simulink model "DroneForwardingSimulation"  (R2022b)
settings: Solver=ode45  StartTime=0.0  StopTime=60  MaxStep=0.2  RelTol=1e-4  AbsTol=1e-4
libraries: slpidlib x2
settings Model: Creator=aless  LastModifiedBy=aless

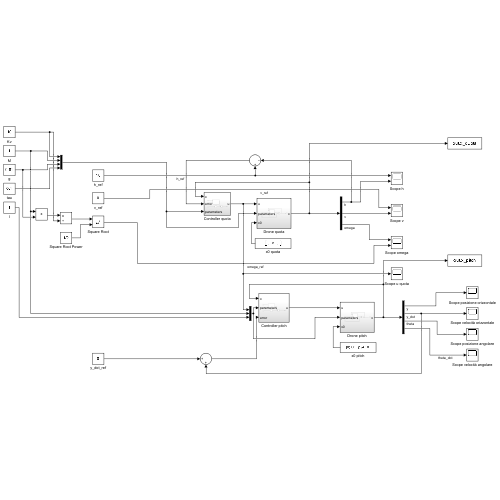
[thumbnail: Simulink's stored preview of the top-level diagram]
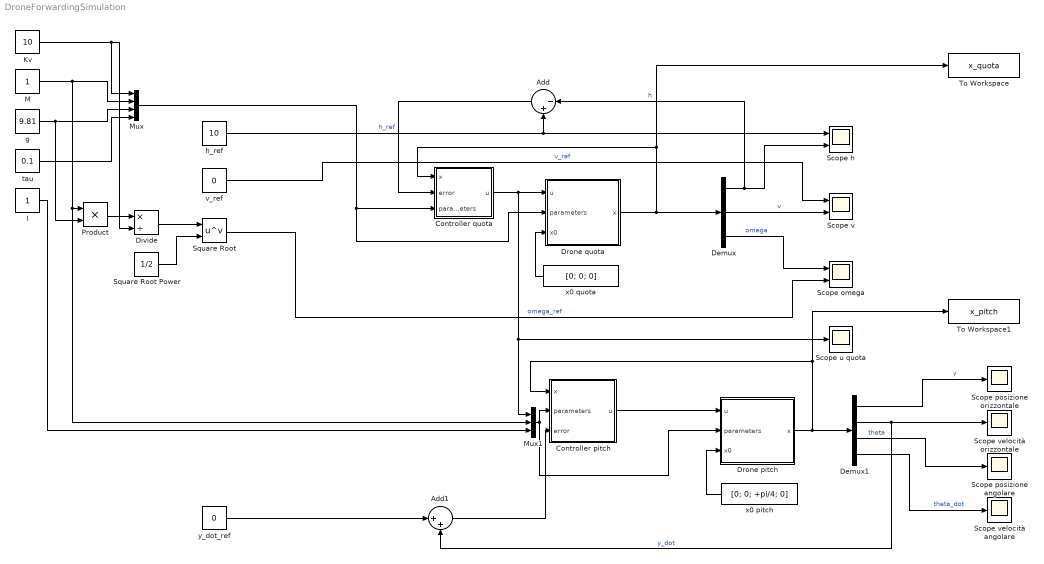
== system DroneForwardingSimulation ==
  Add : Sum  Inputs=|-+
  Add1 : Sum  Inputs=|++
  Controller pitch : Subsystem
  Controller quota : Subsystem
  Demux : Demux  Outputs=3
  Demux1 : Demux
  Divide : Product  Inputs=*/
  Drone pitch : Subsystem
  Drone quota : Subsystem
  I : Constant
  Kv : Constant  Value=10
  M : Constant
  Mux : Mux
  Mux1 : Mux  Inputs=3
  Product : Product
  Scope h : Scope  NumInputPorts=2
  Scope omega : Scope  NumInputPorts=2
  Scope posizione angolare : Scope
  Scope posizione orizzontale : Scope
  Scope u quota : Scope
  Scope v : Scope  NumInputPorts=2
  Scope velocità angolare : Scope
  Scope velocità orizzontale : Scope
  Square Root : Math  Operator=pow
  Square Root Power : Constant  Value=1/2
  To Workspace : ToWorkspace  VariableName=x_quota  SaveFormat=Timeseries  SampleTime=-1
  To Workspace1 : ToWorkspace  VariableName=x_pitch  SaveFormat=Timeseries  SampleTime=-1
  g : Constant  Value=9.81
  h_ref : Constant  Value=10
  tau : Constant  Value=0.1
  v_ref : Constant  Value=0
  x0 pitch : Constant  Value=[0; 0; +pi/4; 0]
  x0 quota : Constant  Value=[0; 0; 0]
  y_dot_ref : Constant  Value=0
  wires:
  Drone quota/1(x) -> To Workspace/1, Controller quota/1(x), Demux/1
  Controller quota/1(u) -> Mux1/1, Scope u quota/1, Drone quota/1(u)
  Demux/1 -> Add/1, Scope h/2  "h"
  g/1 -> Product/2, Mux/3
  M/1 -> Mux1/2, Product/1, Mux/2
  Kv/1 -> Divide/2, Mux/1
  tau/1 -> Mux/4
  Demux/2 -> Scope v/2  "v"
  Demux/3 -> Scope omega/1  "omega"
  x0 quota/1 -> Drone quota/3(x0)
  h_ref/1 -> Scope h/1, Add/2  "h_ref"
  Square Root Power/1 -> Square Root/2
  Product/1 -> Divide/1
  Divide/1 -> Square Root/1
  Square Root/1 -> Scope omega/2  "omega_ref"
  v_ref/1 -> Scope v/1  "v_ref"
  Mux/1 -> Drone quota/2(parameters), Controller quota/3(parameters)
  Add/1 -> Controller quota/2(error)
  Controller pitch/1(u) -> Drone pitch/1(u)
  x0 pitch/1 -> Drone pitch/3(x0)
  Mux1/1 -> Drone pitch/2(parameters), Controller pitch/2(parameters)
  Drone pitch/1(x) -> Demux1/1, To Workspace1/1, Controller pitch/1(x)
  I/1 -> Mux1/3
  Demux1/1 -> Scope posizione orizzontale/1  "y"
  Demux1/2 -> Add1/2, Scope velocità orizzontale/1  "y_dot"
  Demux1/3 -> Scope posizione angolare/1  "theta"
  Demux1/4 -> Scope velocità angolare/1  "theta_dot"
  Add1/1 -> Controller pitch/3(error)
  y_dot_ref/1 -> Add1/1

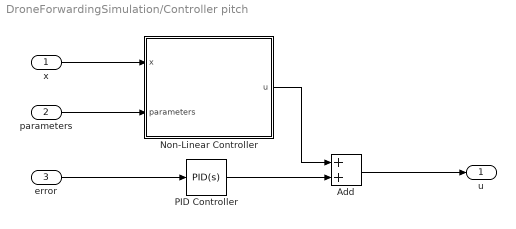
== system DroneForwardingSimulation/Controller pitch ==
  x : Inport
  parameters : Inport  Port=2
  error : Inport  Port=3
  Add : Sum
  Non-Linear Controller : MATLAB Function  TreatAsAtomicUnit=on
  PID Controller : slpidlib/PID Controller  Controller=PID  Form=Parallel  TimeDomain=Continuous-time  UseExternalTs=off  SampleTime=-1  IntegratorMethod=Forward Euler  FilterMethod=Forward Euler  ControllerParametersSource=internal  P=1  I=0.1  UseKiTs=off  D=0  N=100  UseFilter=on  TunerSelectOption=Transfer Function Based (PID Tuner App)  InitialConditionSource=internal  InitialConditionForIntegrator=0  InitialConditionForFilter=0  DifferentiatorICPrevScaledInput=0  ExternalReset=none  TrackingMode=off  Kt=1  LimitOutput=off  SatLimitsSource=internal  UpperSaturationLimit=inf  LowerSaturationLimit=-inf  LinearizeAsGain=on  AntiWindupMode=none  Kb=1  LimitIntegrator=off  UpperIntegratorSaturationLimit=inf  LowerIntegratorSaturationLimit=-inf  POutMin=[]  POutMax=[]  IOutMin=[]  IOutMax=[]  DOutMin=[]  DOutMax=[]  NOutMin=[]  NOutMax=[]  SumOutMin=[]  SumOutMax=[]  SaturationOutMin=[]  SaturationOutMax=[]  PParamMin=[]  PParamMax=[]  IParamMin=[]  IParamMax=[]  DParamMin=[]  DParamMax=[]  NParamMin=[]  NParamMax=[]  KbParamMin=[]  KbParamMax=[]  KtParamMin=[]  KtParamMax=[]  KbOutMin=[]  KbOutMax=[]  KtOutMin=[]  KtOutMax=[]  IntegratorOutMin=[]  IntegratorOutMax=[]  FilterOutMin=[]  FilterOutMax=[]  SumI1OutMin=[]  SumI1OutMax=[]  SumI2OutMin=[]  SumI2OutMax=[]  SumI3OutMin=[]  SumI3OutMax=[]  SumI4OutMin=[]  SumI4OutMax=[]  SumDOutMin=[]  SumDOutMax=[]  DifferentiatorOutMin=[]  DifferentiatorOutMax=[]  FilterDiffOutCoefMin=[]  FilterDiffOutCoefMax=[]  ReciprocalOutMin=[]  ReciprocalOutMax=[]  SumDenOutMin=[]  SumDenOutMax=[]  SumNumOutMin=[]  SumNumOutMax=[]  DivideOutMin=[]  DivideOutMax=[]  UdiffTsProdOutMin=[]  UdiffTsProdOutMax=[]  NTsProdOutMin=[]  NTsProdOutMax=[]  UintegralTsProdOutMin=[]  UintegralTsProdOutMax=[]  UngainTsProdOutMin=[]  UngainTsProdOutMax=[]  ClampingZeroOutDataTypeStr=Inherit: Inherit via back propagation  ClampingZeroOutMin=[]  ClampingZeroOutMax=[]  FilterDenConstantOutDataTypeStr=Inherit: Inherit via back propagation  FilterDenConstantOutMin=[]  FilterDenConstantOutMax=[]  PCopyOutDataTypeStr=Inherit: Inherit via back propagation  PCopyOutMin=[]  PCopyOutMax=[]  NCopyOutDataTypeStr=Inherit: Inherit via back propagation  NCopyOutMin=[]  NCopyOutMax=[]  IntegratorContinuousStateAttributes=''  IntegratorStateMustResolveToSignalObject=off  IntegratorRTWStateStorageClass=Auto  FilterContinuousStateAttributes=''  FilterStateMustResolveToSignalObject=off  FilterRTWStateStorageClass=Auto  ParallelPVariant=InternalParameters  IdealPVariant=Disabled  IVariant=InternalParameters  DVariant=InternalParameters  IntegratorVariant=Continuous  SatVariant=Disabled  AWVariant=Passthrough  PCopyVariant=Disabled  TRVariant=Disabled  FdbkBlocksVariant=Forward  IdealPFdbkVariant=Disabled  SatFdbkVariant=Disabled  DerivativeFilterVariant=ContFilter  NVariant=InternalParameters  NCopyVariant=Disabled  FilterICVariant=InternalICsFilter  IntegratorICVariant=InternalICs  ExternalResetVariant=Disabled  TRSumVariant=Passthrough  SumFdbkVariant=Disabled  SumVariant=Sum_PID  TsampFilterVariant=InternalTs  TsampNgainVariant=Passthrough  TsampIntegralVariant=Passthrough  ExternalSaturationOutDataTypeStr=Inherit: Same as second input
  u : Outport
  wires:
  parameters/1 -> Non-Linear Controller/2(parameters)
  x/1 -> Non-Linear Controller/1(x)
  error/1 -> PID Controller/1
  Non-Linear Controller/1(u) -> Add/1
  Add/1 -> u/1
  PID Controller/1 -> Add/2

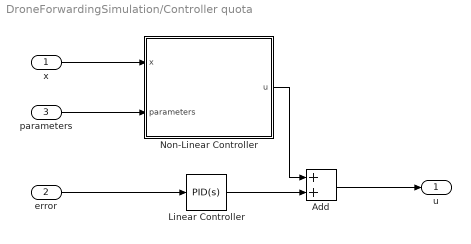
== system DroneForwardingSimulation/Controller quota ==
  x : Inport
  error : Inport  Port=2
  parameters : Inport  Port=3
  Add : Sum
  Linear Controller : slpidlib/PID Controller  Controller=PID  Form=Parallel  TimeDomain=Continuous-time  UseExternalTs=off  SampleTime=-1  IntegratorMethod=Forward Euler  FilterMethod=Forward Euler  ControllerParametersSource=internal  P=10  I=1  UseKiTs=off  D=0  N=100  UseFilter=on  TunerSelectOption=Transfer Function Based (PID Tuner App)  InitialConditionSource=internal  InitialConditionForIntegrator=0  InitialConditionForFilter=0  DifferentiatorICPrevScaledInput=0  ExternalReset=none  TrackingMode=off  Kt=1  LimitOutput=off  SatLimitsSource=internal  UpperSaturationLimit=inf  LowerSaturationLimit=-inf  LinearizeAsGain=on  AntiWindupMode=none  Kb=1  LimitIntegrator=off  UpperIntegratorSaturationLimit=inf  LowerIntegratorSaturationLimit=-inf  POutMin=[]  POutMax=[]  IOutMin=[]  IOutMax=[]  DOutMin=[]  DOutMax=[]  NOutMin=[]  NOutMax=[]  SumOutMin=[]  SumOutMax=[]  SaturationOutMin=[]  SaturationOutMax=[]  PParamMin=[]  PParamMax=[]  IParamMin=[]  IParamMax=[]  DParamMin=[]  DParamMax=[]  NParamMin=[]  NParamMax=[]  KbParamMin=[]  KbParamMax=[]  KtParamMin=[]  KtParamMax=[]  KbOutMin=[]  KbOutMax=[]  KtOutMin=[]  KtOutMax=[]  IntegratorOutMin=[]  IntegratorOutMax=[]  FilterOutMin=[]  FilterOutMax=[]  SumI1OutMin=[]  SumI1OutMax=[]  SumI2OutMin=[]  SumI2OutMax=[]  SumI3OutMin=[]  SumI3OutMax=[]  SumI4OutMin=[]  SumI4OutMax=[]  SumDOutMin=[]  SumDOutMax=[]  DifferentiatorOutMin=[]  DifferentiatorOutMax=[]  FilterDiffOutCoefMin=[]  FilterDiffOutCoefMax=[]  ReciprocalOutMin=[]  ReciprocalOutMax=[]  SumDenOutMin=[]  SumDenOutMax=[]  SumNumOutMin=[]  SumNumOutMax=[]  DivideOutMin=[]  DivideOutMax=[]  UdiffTsProdOutMin=[]  UdiffTsProdOutMax=[]  NTsProdOutMin=[]  NTsProdOutMax=[]  UintegralTsProdOutMin=[]  UintegralTsProdOutMax=[]  UngainTsProdOutMin=[]  UngainTsProdOutMax=[]  ClampingZeroOutDataTypeStr=Inherit: Inherit via back propagation  ClampingZeroOutMin=[]  ClampingZeroOutMax=[]  FilterDenConstantOutDataTypeStr=Inherit: Inherit via back propagation  FilterDenConstantOutMin=[]  FilterDenConstantOutMax=[]  PCopyOutDataTypeStr=Inherit: Inherit via back propagation  PCopyOutMin=[]  PCopyOutMax=[]  NCopyOutDataTypeStr=Inherit: Inherit via back propagation  NCopyOutMin=[]  NCopyOutMax=[]  IntegratorContinuousStateAttributes=''  IntegratorStateMustResolveToSignalObject=off  IntegratorRTWStateStorageClass=Auto  FilterContinuousStateAttributes=''  FilterStateMustResolveToSignalObject=off  FilterRTWStateStorageClass=Auto  ParallelPVariant=InternalParameters  IdealPVariant=Disabled  IVariant=InternalParameters  DVariant=InternalParameters  IntegratorVariant=Continuous  SatVariant=Disabled  AWVariant=Passthrough  PCopyVariant=Disabled  TRVariant=Disabled  FdbkBlocksVariant=Forward  IdealPFdbkVariant=Disabled  SatFdbkVariant=Disabled  DerivativeFilterVariant=ContFilter  NVariant=InternalParameters  NCopyVariant=Disabled  FilterICVariant=InternalICsFilter  IntegratorICVariant=InternalICs  ExternalResetVariant=Disabled  TRSumVariant=Passthrough  SumFdbkVariant=Disabled  SumVariant=Sum_PID  TsampFilterVariant=InternalTs  TsampNgainVariant=Passthrough  TsampIntegralVariant=Passthrough  ExternalSaturationOutDataTypeStr=Inherit: Same as second input
  Non-Linear Controller : MATLAB Function  TreatAsAtomicUnit=on
  u : Outport
  wires:
  Non-Linear Controller/1(u) -> Add/1
  parameters/1 -> Non-Linear Controller/2(parameters)
  x/1 -> Non-Linear Controller/1(x)
  error/1 -> Linear Controller/1
  Add/1 -> u/1
  Linear Controller/1 -> Add/2

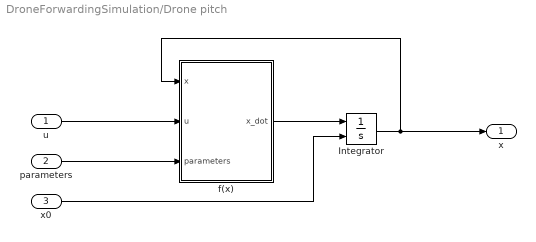
== system DroneForwardingSimulation/Drone pitch ==
  u : Inport
  parameters : Inport  Port=2
  x0 : Inport  Port=3
  Integrator : Integrator  InitialConditionSource=external
  f(x) : MATLAB Function  TreatAsAtomicUnit=on
  x : Outport
  wires:
  Integrator/1 -> x/1, f(x)/1(x)
  f(x)/1(x_dot) -> Integrator/1
  u/1 -> f(x)/2(u)
  parameters/1 -> f(x)/3(parameters)
  x0/1 -> Integrator/2

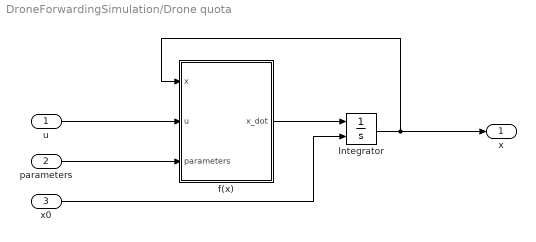
== system DroneForwardingSimulation/Drone quota ==
  u : Inport
  parameters : Inport  Port=2
  x0 : Inport  Port=3
  Integrator : Integrator  InitialConditionSource=external
  f(x) : MATLAB Function  TreatAsAtomicUnit=on
  x : Outport
  wires:
  Integrator/1 -> x/1, f(x)/1(x)
  f(x)/1(x_dot) -> Integrator/1
  u/1 -> f(x)/2(u)
  parameters/1 -> f(x)/3(parameters)
  x0/1 -> Integrator/2

== matlab function DroneForwardingSimulation/Controller quota/Non-Linear Controller ==
  data: x input; u output; parameters input
function u = fcn(x, parameters)

    Kv =    parameters(1);
    M =     parameters(2);
    g =     parameters(3);
    tau =   parameters(4);

    u0 = sqrt(g*M/Kv);

    u1 = - (x(3) + (x(2) + tau * Kv/(2*M) * x(3)^2) * tau * Kv/M * x(3)) * 1/tau;

    u2 = - (x(2) + (x(1) + tau^2 * Kv/(4*M) * x(3)^2) * tau^2 * Kv/(2*M) * x(3)) * 1/tau;

    u = u0 + u1 + u2;

end

== matlab function DroneForwardingSimulation/Drone quota/f(x) ==
  data: x input; u input; x_dot output; parameters input
function x_dot = fcn(x, u, parameters)

    Kv =    parameters(1);
    M =     parameters(2);
    g =     parameters(3);
    tau =   parameters(4);

    x_dot = [x(2);
            (Kv/M)*x(3)^2 - g;
            (-x(3)+u)/tau];

end

== matlab function DroneForwardingSimulation/Drone pitch/f(x) ==
  data: x input; u input; x_dot output; parameters input
function x_dot = fcn(x, u, parameters)

    T =     parameters(1);
    M =     parameters(2);
    I =     parameters(3);

    x_dot = [+x(2);
             -T/M * sin(x(3));
             +x(4);
             1/I * u];

end

== matlab function DroneForwardingSimulation/Controller pitch/Non-Linear Controller ==
  data: x input; u output; parameters input
function u = fcn(x, parameters)

    T =     parameters(1);
    M =     parameters(2);
    I =     parameters(3);

    u0 = - x(4);

    u1 = - (x(4) + (x(3) + I*x(4)) * I) * 1/I;

    % u2 = - (x(3) - (x(2) + T/M * (cos(I*x(4)) / x(4))) * T/M * (sin(I*x(4))*x(4) + cos(I*x(4)))/(x(4)^2)) * 1/I;

    u = u0 + u1;

end
